simulink model "VendingMachine"  (R2020b)
settings: Solver=ode2  StartTime=0.0  StopTime=500  RelTol=1e-3
settings Model: Creator=Sourav Kumar  LastModifiedBy=Sourav Kumar
settings DataIOCC: SaveFormat=Array
settings DebuggingCC: SolverPrmCheckMsg=warning  StateNameClashWarn=warning
settings ModelReferenceCC: PropagateSignalLabelsOutOfModel=off
settings SFSimCC: SimParseCustomCode=off

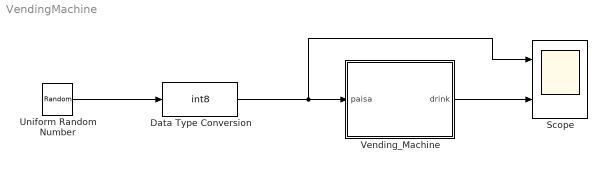
== system VendingMachine ==
  Data Type Conversion : DataTypeConversion  OutDataTypeStr=int8  RndMeth=Nearest  SaturateOnIntegerOverflow=on
  Scope : Scope  NumInputPorts=2
  Uniform Random Number : UniformRandomNumber  Minimum=0  Maximum=5  Seed=250  SampleTime=10
  Vending_Machine : Stateflow chart  TreatAsAtomicUnit=on
  wires:
  Uniform Random Number/1 -> Data Type Conversion/1
  Data Type Conversion/1 -> Scope/1, Vending_Machine/1(paisa)
  Vending_Machine/1(drink) -> Scope/2

== stateflow chart VendingMachine/Vending_Machine ==
  settings: stateMachineType=MEALY_MACHINE  initializeOutput=1
  state got_0
  state got_nickel
  state got_dime
  (default) -> got_0
  got_0 -> got_nickel [order 1] : [paisa==1]{drink=0}
  got_nickel -> got_0 [order 2] : [paisa==2]{drink=1}
  got_dime -> got_0 [order 1] : [paisa==1]{drink=1}
  got_0 -> got_dime [order 2] : [paisa==2]{drink=0}
  got_nickel -> got_dime [order 1] : [paisa==1]{drink=0}
  got_dime -> got_nickel [order 2] : [paisa==2]{drink=1}
  data: paisa input; drink output double
